simulink model "tempreture_trans"  (R2018a)
settings: Solver=VariableStepAuto  StartTime=0.0  StopTime=10  RelTol=1e-3
settings Model: Creator=Li Gen  LastModifiedBy=Li Gen

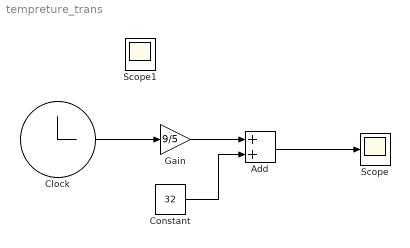
== system tempreture_trans ==
  Add : Sum
  Clock : Clock
      settings: Decimation=100
  Constant : Constant  Value=32
  Gain : Gain  Gain=9/5
  Scope : Scope
  Scope1 : Scope
  wires:
  Clock/1 -> Gain/1
  Gain/1 -> Add/1
  Constant/1 -> Add/2
  Add/1 -> Scope/1
